simulink model "Fuchs_FDFR_simulink_nonlinear"  (R2024a)
settings: Solver=ode4  StartTime=0.0  StopTime=300  FixedStep=0.02  RelTol=1e-3
libraries: vrlib x1
(part 1 of 3)
settings Model: Creator=finnf  LastModifiedBy=finnf

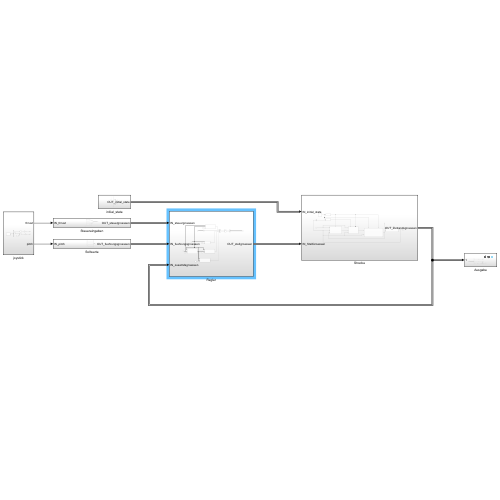
[thumbnail: Simulink's stored preview of the top-level diagram]
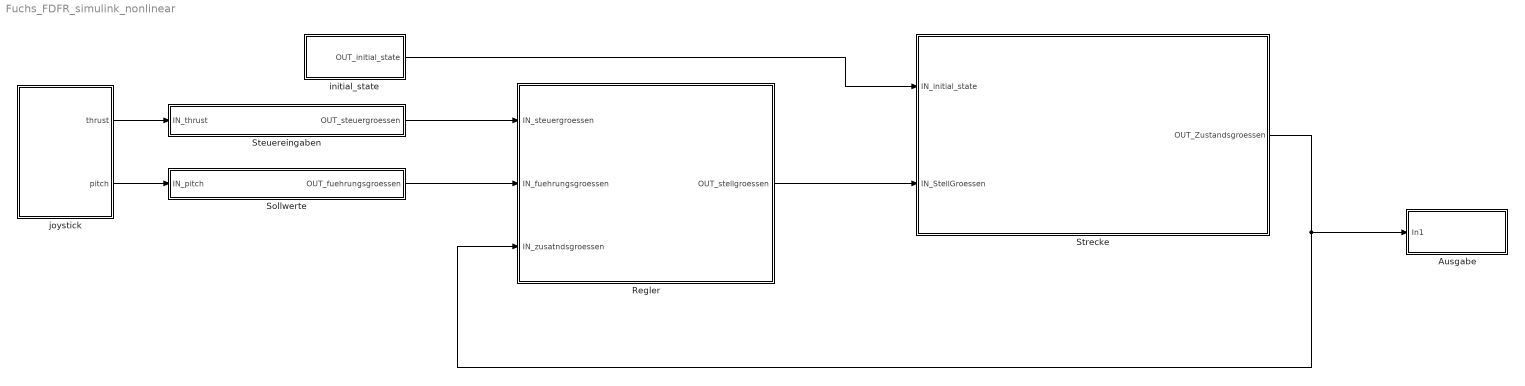
== system Fuchs_FDFR_simulink_nonlinear ==
  Ausgabe : Subsystem
  Regler : Subsystem
  Sollwerte : Subsystem
  Steuereingaben : Subsystem
  Strecke : Subsystem
  initial_state : Subsystem
  joystick : Subsystem
  wires:
  Strecke/1(OUT_Zustandsgroessen) -> Ausgabe/1(In1), Regler/3(IN_zusatndsgroessen)
  Regler/1(OUT_stellgroessen) -> Strecke/2(IN_StellGroessen)
  Sollwerte/1(OUT_fuehrungsgroessen) -> Regler/2(IN_fuehrungsgroessen)
  Steuereingaben/1(OUT_steuergroessen) -> Regler/1(IN_steuergroessen)
  initial_state/1(OUT_initial_state) -> Strecke/1(IN_initial_state)
  joystick/2(pitch) -> Sollwerte/1(IN_pitch)
  joystick/1(thrust) -> Steuereingaben/1(IN_thrust)

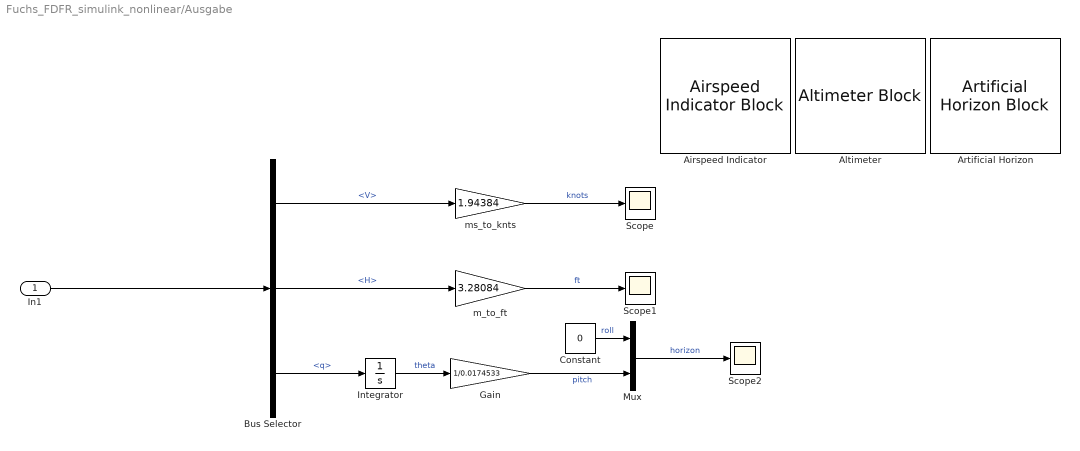
== system Fuchs_FDFR_simulink_nonlinear/Ausgabe ==
  In1 : Inport
  Airspeed Indicator : AirspeedIndicatorBlock  ScaleMin=80  ScaleMax=800
  Altimeter : AltimeterBlock
  Artificial Horizon : ArtificialHorizonBlock
  Bus Selector : BusSelector  OutputSignals=V,H,q
  Constant : Constant  Value=0
  Gain : Gain  Gain=1/0.0174533
  Integrator : Integrator
  Mux : Mux  Inputs=2
  Scope : Scope
  Scope1 : Scope
  Scope2 : Scope
  m_to_ft : Gain  Gain=3.28084
  ms_to_knts : Gain  Gain=1.94384
  wires:
  In1/1 -> Bus Selector/1
  Bus Selector/1 -> ms_to_knts/1  "<V>"
  Bus Selector/2 -> m_to_ft/1  "<H>"
  Bus Selector/3 -> Integrator/1  "<q>"
  Integrator/1 -> Gain/1  "theta"
  Gain/1 -> Mux/2  "pitch"
  Constant/1 -> Mux/1  "roll"
  ms_to_knts/1 -> Scope/1  "knots"
  m_to_ft/1 -> Scope1/1  "ft"
  Mux/1 -> Scope2/1  "horizon"

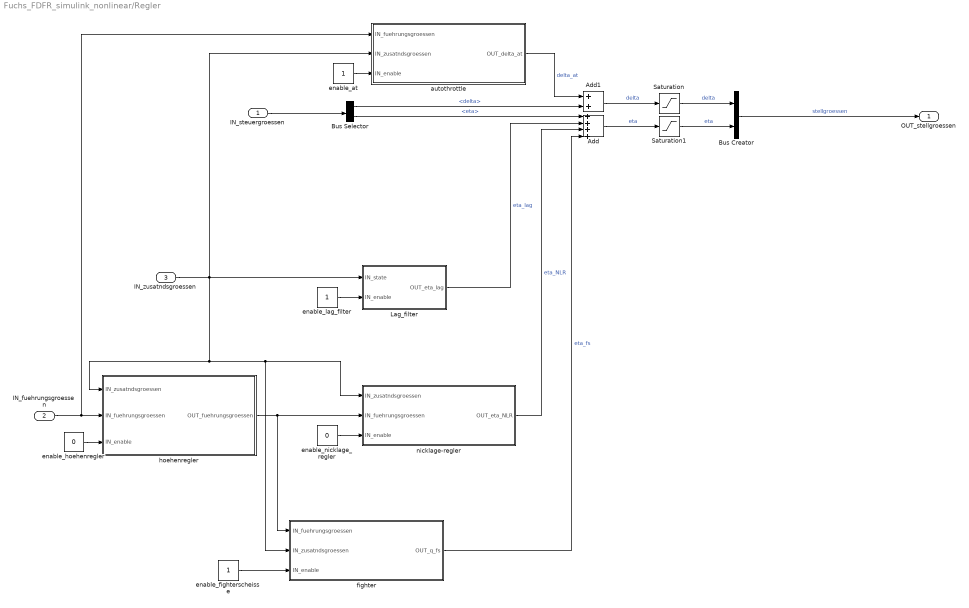
== system Fuchs_FDFR_simulink_nonlinear/Regler ==
  IN_steuergroessen : Inport
  IN_fuehrungsgroessen : Inport  Port=2
  IN_zusatndsgroessen : Inport  Port=3
  Add : Sum  Inputs=++++
  Add1 : Sum
  Bus Creator : BusCreator  Inputs=2
  Bus Selector : BusSelector  OutputSignals=delta,eta
  Lag_filter : Subsystem
  Saturation : Saturate  UpperLimit=1  LowerLimit=0
  Saturation1 : Saturate  UpperLimit=20*pi/180  LowerLimit=-20*pi/180
  autothrottle : Subsystem
  enable_at : Constant
  enable_fighterscheisse : Constant
  enable_hoehenregler : Constant  Value=0
  enable_lag_filter : Constant
  enable_nicklage_regler : Constant  Value=0
  fighter : Subsystem
  hoehenregler : Subsystem
  nicklage-regler : Subsystem
  OUT_stellgroessen : Outport
  wires:
  Bus Creator/1 -> OUT_stellgroessen/1  "stellgroessen"
  Bus Selector/1 -> Add1/2  "<delta>"
  IN_steuergroessen/1 -> Bus Selector/1
  IN_zusatndsgroessen/1 -> Lag_filter/1(IN_state), nicklage-regler/1(IN_zusatndsgroessen), fighter/2(IN_zusatndsgroessen), hoehenregler/1(IN_zusatndsgroessen), autothrottle/2(IN_zusatndsgroessen)
  enable_lag_filter/1 -> Lag_filter/2(IN_enable)
  Lag_filter/1(OUT_eta_lag) -> Add/2  "eta_lag"
  Add/1 -> Saturation1/1  "eta"
  Bus Selector/2 -> Add/1  "<eta>"
  nicklage-regler/1(OUT_eta_NLR) -> Add/3  "eta_NLR"
  IN_fuehrungsgroessen/1 -> autothrottle/1(IN_fuehrungsgroessen), hoehenregler/2(IN_fuehrungsgroessen)
  enable_nicklage_regler/1 -> nicklage-regler/3(IN_enable)
  hoehenregler/1(OUT_fuehrungsgroessen) -> fighter/1(IN_fuehrungsgroessen), nicklage-regler/2(IN_fuehrungsgroessen)
  enable_hoehenregler/1 -> hoehenregler/3(IN_enable)
  Add1/1 -> Saturation/1  "delta"
  autothrottle/1(OUT_delta_at) -> Add1/1  "delta_at"
  enable_at/1 -> autothrottle/3(IN_enable)
  Saturation/1 -> Bus Creator/1  "delta"
  Saturation1/1 -> Bus Creator/2  "eta"
  enable_fighterscheisse/1 -> fighter/3(IN_enable)
  fighter/1(OUT_q_fs) -> Add/4  "eta_fs"

== system Fuchs_FDFR_simulink_nonlinear/Sollwerte ==
  IN_pitch : Inport
  Bus Creator : BusCreator  Inputs=4
  alt_m : Constant  Value=9750
  theta : Constant  Value=0
  vel_ms : Constant  Value=265
  OUT_fuehrungsgroessen : Outport
  wires:
  Bus Creator/1 -> OUT_fuehrungsgroessen/1
  theta/1 -> Bus Creator/1  "theta_c"
  alt_m/1 -> Bus Creator/2  "alt_c"
  vel_ms/1 -> Bus Creator/3  "vel_c"
  IN_pitch/1 -> Bus Creator/4  "q_c"

== system Fuchs_FDFR_simulink_nonlinear/Steuereingaben ==
  IN_thrust : Inport
  Add : Sum
  Add1 : Sum  Inputs=+++
  Bus Creator : BusCreator  Inputs=2
  delta_dist : Constant  Value=0
  delta_ref trim: 0.378775311827620 : Constant  Value=0
  eta_dist : Constant  Value=0
  "eta_ref trim:0.098372238870606 " : Constant  Value=0
  OUT_steuergroessen : Outport
  wires:
  Bus Creator/1 -> OUT_steuergroessen/1  "steuergroessen"
  "eta_ref trim:0.098372238870606 "/1 -> Add/2  "eta"
  delta_ref trim: 0.378775311827620/1 -> Add1/1  "delta"
  Add/1 -> Bus Creator/1  "eta"
  eta_dist/1 -> Add/1  "eta"
  delta_dist/1 -> Add1/2  "delta"
  Add1/1 -> Bus Creator/2  "delta"
  IN_thrust/1 -> Add1/3

== system Fuchs_FDFR_simulink_nonlinear/Strecke ==
  IN_initial_state : Inport
  IN_StellGroessen : Inport  Port=2
  Beiwerte : Subsystem
      settings: PortSchema="{\"entries\":[{\"content\":{\"sides\":[{\"content\":{\"connectorIds\":[\"In1\",\"In2\",\"In3\"]},\"type\":\"ConnectorPlacement.EquallySpacedRectSide\",\"uuid\":\"da868e00-0983-4992-b3a2-0cb597f348b4\"},{\"content\":{\"connectorIds\":[\"Out1\"],\"side\":\"RIGHT\"},\"type\":\"ConnectorPlacement.EquallySpacedRectSide\",\"uuid\":\"845dd281-7800-4d97-986c-16221190292f\"},{\"content\":{\"connectorIds\":[\"In4\"],\"side\":\"TOP\"},\"type\":\"ConnectorPlacement.EquallySpacedRectSide\",\"uuid\":\"2d5432b3-412d-4b60-8ef0-e3903cbc0053\"}]},\"type\":\"ConnectorPlacement.EquallySpacedConnector\",\"uuid\":\"2421fdf9-bf27-4e89-90d1-e2d9d3a90679\"}],\"packageUris\":[\"http://schema.mathworks.com/mf0/Connector/R2020b\"],\"version\":\"1.0\"}"
  Bus Selector : BusSelector  OutputSignals=H
  DGL : Subsystem
      settings: PortSchema="{\"entries\":[{\"content\":{\"sides\":[{\"content\":{\"connectorIds\":[\"In1\",\"In2\"]},\"type\":\"ConnectorPlacement.EquallySpacedRectSide\",\"uuid\":\"da868e00-0983-4992-b3a2-0cb597f348b4\"},{\"content\":{\"connectorIds\":[\"Out1\"],\"side\":\"RIGHT\"},\"type\":\"ConnectorPlacement.EquallySpacedRectSide\",\"uuid\":\"845dd281-7800-4d97-986c-16221190292f\"},{\"content\":{\"connectorIds\":[\"In3\",\"In4\"],\"side\":\"TOP\"},\"type\":\"ConnectorPlacement.EquallySpacedRectSide\",\"uuid\":\"2d5432b3-412d-4b60-8ef0-e3903cbc0053\"}]},\"type\":\"ConnectorPlacement.EquallySpacedConnector\",\"uuid\":\"2421fdf9-bf27-4e89-90d1-e2d9d3a90679\"}],\"packageUris\":[\"http://schema.mathworks.com/mf0/Connector/R2020b\"],\"version\":\"1.0\"}"
  Integratorsys : Subsystem
  Kraefte_Momente : Subsystem
      settings: PortSchema="{\"entries\":[{\"content\":{\"sides\":[{\"content\":{\"connectorIds\":[\"In1\",\"In2\",\"In3\"]},\"type\":\"ConnectorPlacement.EquallySpacedRectSide\",\"uuid\":\"7b0f2669-d239-479f-ac51-e28c31c4b0e7\"},{\"content\":{\"connectorIds\":[\"Out1\"],\"side\":\"RIGHT\"},\"type\":\"ConnectorPlacement.EquallySpacedRectSide\",\"uuid\":\"e76e6a99-f945-4a89-9fd0-954498cc0474\"},{\"content\":{\"connectorIds\":[\"In4\",\"In5\"],\"side\":\"TOP\"},\"type\":\"ConnectorPlacement.EquallySpacedRectSide\",\"uuid\":\"f108f290-1f7b-41fa-80e9-36849535a7ac\"}]},\"type\":\"ConnectorPlacement.EquallySpacedConnector\",\"uuid\":\"a57fc054-3292-469b-8cca-8ca2c9194743\"}],\"packageUris\":[\"http://schema.mathworks.com/mf0/Connector/R2020b\"],\"version\":\"1.0\"}"
  get_rho_of_alt1 : Subsystem
  init_ac : Subsystem
  init_env : Subsystem
  OUT_Zustandsgroessen : Outport
  wires:
  Kraefte_Momente/1(OUT_kraefte_momente) -> DGL/1(IN_kraefte_momente)  "kraefte_momente"
  Beiwerte/1(OUT_beiwerte) -> Kraefte_Momente/2(IN_beiwerte)  "beiwerte"
  IN_StellGroessen/1 -> Kraefte_Momente/1(IN_steuereingaben), Beiwerte/1(IN_Steuereigaben)
  Integratorsys/1(OUT_zustandsgroessen) -> Bus Selector/1, Beiwerte/2(IN_Zustandsgroessen), Kraefte_Momente/3(IN_zustandsgroessen), DGL/2(IN_zustandsgroessen), OUT_Zustandsgroessen/1  "zustandsgroessen"
  init_env/1(env) -> get_rho_of_alt1/1(IN_env), DGL/3(IN_enviroment), init_ac/1(in_env)  "env"
  Bus Selector/1 -> get_rho_of_alt1/2(IN_alt_m)  "<H>"
  init_ac/1(ac) -> DGL/4(IN_aircraft), Kraefte_Momente/5(IN_ac), Beiwerte/4(IN_ac)  "ac"
  get_rho_of_alt1/1(rho) -> Kraefte_Momente/4(IN_rho)  "rho"
  IN_initial_state/1 -> Integratorsys/1(IN_initial_state)
  DGL/1(OUT_zustandsgroessen_dot) -> Beiwerte/3(IN_zustandsgroessen_dot), Integratorsys/2(IN_zustandsgroessen_dot)

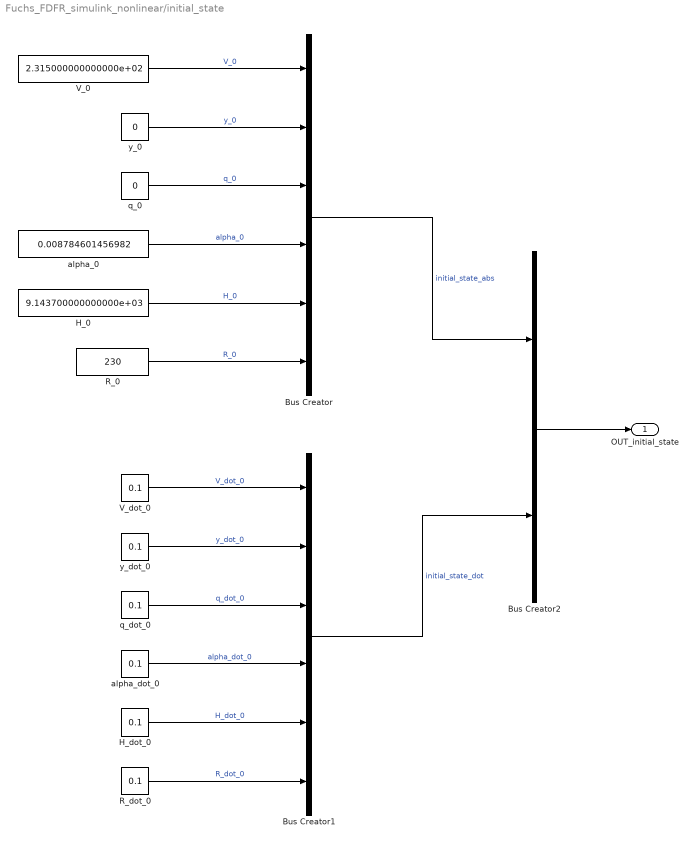
== system Fuchs_FDFR_simulink_nonlinear/initial_state ==
  Bus Creator : BusCreator  Inputs=6
  Bus Creator1 : BusCreator  Inputs=6
  Bus Creator2 : BusCreator  Inputs=2
  H_0 : Constant  Value=9.143700000000000e+03
  H_dot_0 : Constant  Value=0.1
  R_0 : Constant  Value=230
  R_dot_0 : Constant  Value=0.1
  V_0 : Constant  Value=2.315000000000000e+02
  V_dot_0 : Constant  Value=0.1
  alpha_0 : Constant  Value=0.008784601456982
  alpha_dot_0 : Constant  Value=0.1
  q_0 : Constant  Value=0
  q_dot_0 : Constant  Value=0.1
  y_0 : Constant  Value=0
  y_dot_0 : Constant  Value=0.1
  OUT_initial_state : Outport
  wires:
  Bus Creator/1 -> Bus Creator2/1  "initial_state_abs"
  V_0/1 -> Bus Creator/1  "V_0"
  y_0/1 -> Bus Creator/2  "y_0"
  q_0/1 -> Bus Creator/3  "q_0"
  alpha_0/1 -> Bus Creator/4  "alpha_0"
  H_0/1 -> Bus Creator/5  "H_0"
  R_0/1 -> Bus Creator/6  "R_0"
  y_dot_0/1 -> Bus Creator1/2  "y_dot_0"
  q_dot_0/1 -> Bus Creator1/3  "q_dot_0"
  H_dot_0/1 -> Bus Creator1/5  "H_dot_0"
  R_dot_0/1 -> Bus Creator1/6  "R_dot_0"
  V_dot_0/1 -> Bus Creator1/1  "V_dot_0"
  alpha_dot_0/1 -> Bus Creator1/4  "alpha_dot_0"
  Bus Creator1/1 -> Bus Creator2/2  "initial_state_dot"
  Bus Creator2/1 -> OUT_initial_state/1

== system Fuchs_FDFR_simulink_nonlinear/joystick ==
  Add : Sum  Inputs=-+
  Constant : Constant
  Dead Zone : DeadZone  LowerValue=-0.1  UpperValue=0.1
  Demux : Demux  Outputs=7
  Gain : Gain  Gain=0.5
  Gain1 : Gain
  Joystick Input : vrlib/Joystick Input  joyid=1  adjustports=on  forcefeed=off
  thrust : Outport
  pitch : Outport  Port=2
  wires:
  Joystick Input/1 -> Demux/1
  Demux/3 -> Add/1  "thrust"
  Demux/2 -> Dead Zone/1  "pitch"
  Add/1 -> Gain/1  "thrust_c"
  Constant/1 -> Add/2
  Gain/1 -> thrust/1  "thrust_c"
  Dead Zone/1 -> Gain1/1
  Gain1/1 -> pitch/1
